simulink model "modulation"  (R2018a)
settings: Solver=VariableStepAuto  StartTime=0.0  StopTime=10.0  RelTol=1e-3
settings Model: Creator=Varad  LastModifiedBy=Varad

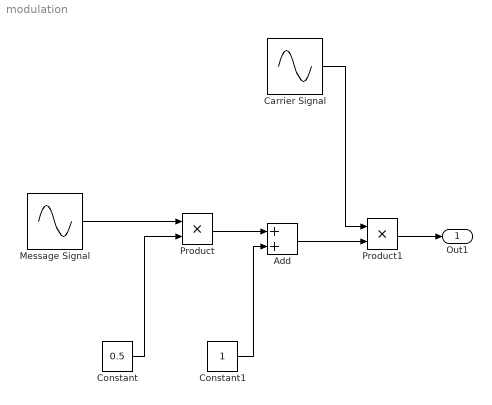
== system modulation ==
  Add : Sum
  Carrier Signal : Sin  Frequency=2*pi*250/2000  SampleTime=0
  Constant : Constant  Value=0.5
  Constant1 : Constant
  "Message Signal " : Sin  Frequency=2*pi*5/2000  Phase=pi/2  SampleTime=0
  Product : Product
  Product1 : Product
  Out1 : Outport
  wires:
  "Message Signal "/1 -> Product/1
  Constant/1 -> Product/2
  Product/1 -> Add/1
  Constant1/1 -> Add/2
  Add/1 -> Product1/2
  Carrier Signal/1 -> Product1/1
  Product1/1 -> Out1/1
